simulink model "TCP"  (R2022b)
settings: Solver=FixedStepAuto  StartTime=0.0  StopTime=50000000  FixedStep=1  RelTol=1e-3
libraries: simulink x9
settings Model: Creator=yuzehong  LastModifiedBy=程一帆
settings OptimizationCC: DefaultParameterBehavior=Inlined  DefaultUnderspecifiedDataType=single  BufferReuse=off  GlobalBufferReuse=off  ExpressionFolding=off  EnableMemcpy=off  PassReuseOutputArgsAs=Individual arguments  OptimizeDataStoreBuffers=off  BusAssignmentInplaceUpdate=off  OptimizationLevel=level0  EfficientTunableParamExpr=on
settings DebuggingCC: ParameterTunabilityLossMsg=error  UnconnectedInputMsg=warning  UnconnectedOutputMsg=warning  UnconnectedLineMsg=warning
settings ModelReferenceCC: EnableRefExpFcnMdlSchedulingChecks=on
settings SFSimCC: MATLABDynamicMemAlloc=off
settings RTWCC: Description=Embedded Coder  SystemTargetFile=ert.tlc  GenCodeOnly=on  TemplateMakefile=ert_default_tmf  DLArmComputeVersion=19.05
settings CodeAppCC: ForceParamTrailComments=on  IgnoreCustomStorageClasses=off  OperatorAnnotations=on  SimulinkDataObjDesc=on  SFDataObjDesc=on  InsertBlockDesc=on
settings ERTTargetCC: TargetLangStandard=C99 (ISO)  GenerateSampleERTMain=on  CodeInterfacePackaging=Reusable function  InlinedParameterPlacement=NonHierarchical  ERTCustomFileTemplate=example_file_process.tlc
settings ConfigComp: DVMaxProcessTime=3600  DVTestSuiteOptimization=Auto  DVDetectOutOfBounds=on  DVSaveHarnessModel=on  DVModelReferenceHarness=on

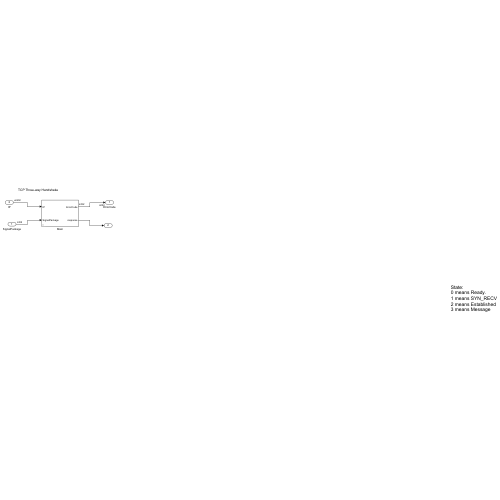
[thumbnail: Simulink's stored preview of the top-level diagram]
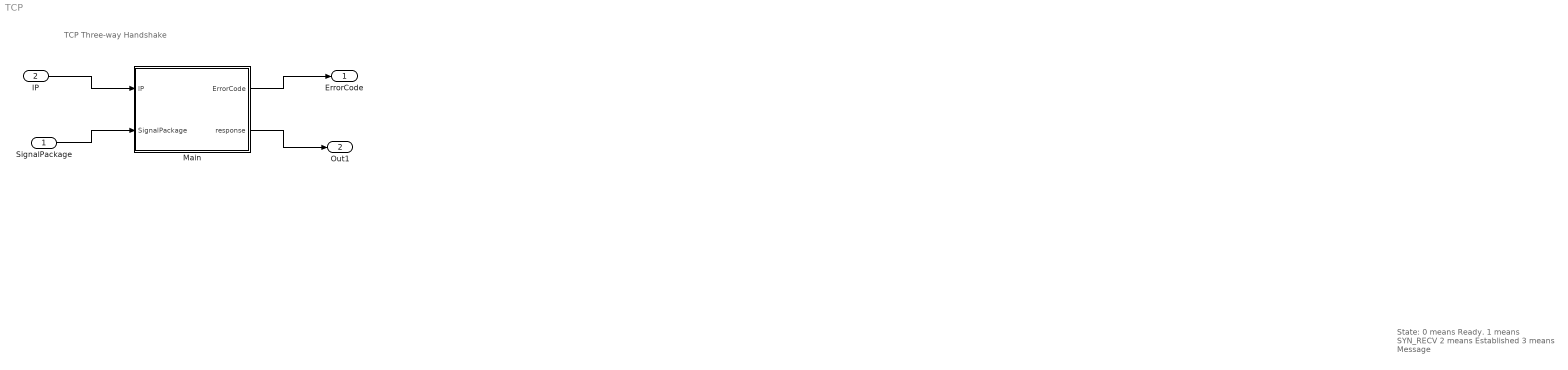
== system TCP ==
  note: TCP Three-way Handshake
  note: State:
      | 0 means Ready.
      | 1 means SYN_RECV
      | 2 means Established
      | 3 means Message
  SignalPackage : Inport  OutDataTypeStr=int32  PortDimensions=1
  IP : Inport  Port=2  OutDataTypeStr=uint32
  Main : Subsystem  mask{Len=16}
      mask DialogControl ParameterGroupVar Prompt: 参数
  ErrorCode : Outport  OutDataTypeStr=int32
  Out1 : Outport  Port=2
  wires:
  IP/1 -> Main/1(IP)
  SignalPackage/1 -> Main/2(SignalPackage)
  Main/1(ErrorCode) -> ErrorCode/1
  Main/2(response) -> Out1/1

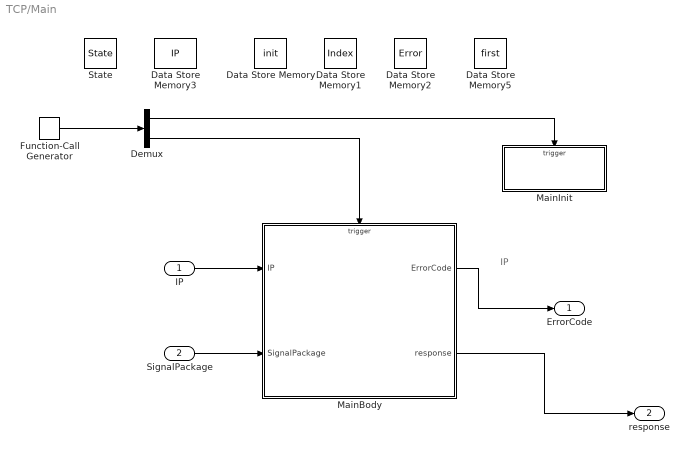
== system TCP/Main ==
  note: IP
  IP : Inport
  SignalPackage : Inport  Port=2
  Data Store Memory : DataStoreMemory  DataStoreName=init  WriteAfterWriteMsg=warning  ShowAdditionalParam=off  OutDataTypeStr=int8
  Data Store Memory1 : DataStoreMemory  DataStoreName=Index  WriteAfterWriteMsg=warning  InitialValue=-1  ShowAdditionalParam=off  OutDataTypeStr=int32
  Data Store Memory2 : DataStoreMemory  DataStoreName=Error  WriteAfterWriteMsg=warning  ShowAdditionalParam=off  OutDataTypeStr=int32
  Data Store Memory3 : DataStoreMemory  DataStoreName=IP  WriteAfterWriteMsg=warning  ShowAdditionalParam=off  OutDataTypeStr=uint32  Dimensions=Len
  Data Store Memory5 : DataStoreMemory  DataStoreName=first  WriteAfterWriteMsg=warning  ShowAdditionalParam=off  OutDataTypeStr=int32
  Demux : Demux  Outputs=2
  Function-Call Generator : simulink/Ports & Subsystems/Function-Call Generator  sample_time=1  numberOfIterations=1  DisallowWideOutput=off
  MainBody : Subsystem  TreatAsAtomicUnit=on
  MainInit : Subsystem  TreatAsAtomicUnit=on
  State : DataStoreMemory  DataStoreName=State  WriteAfterWriteMsg=warning  ShowAdditionalParam=off  OutDataTypeStr=int32  Dimensions=Len
  ErrorCode : Outport  OutDataTypeStr=int32
  response : Outport  Port=2
  wires:
  SignalPackage/1 -> MainBody/2(SignalPackage)
  Function-Call Generator/1 -> Demux/1
  Demux/1 -> MainInit/Trigger
  IP/1 -> MainBody/1(IP)
  MainBody/1(ErrorCode) -> ErrorCode/1
  Demux/2 -> MainBody/Trigger
  MainBody/2(response) -> response/1

== system TCP/Main/MainBody ==
  note: Process IP address.
  note: IP Address cannot be zero
  note: Process Data Package.
  IP : Inport
  SignalPackage : Inport  Port=2
  function : TriggerPort  TriggerType=function-call  VariantControl=(inherit)
  Process : Subsystem
  ErrorCode : Outport  OutDataTypeStr=int32
  response : Outport  Port=2
  wires:
  IP/1 -> Process/1(IP)
  SignalPackage/1 -> Process/2(SignalPackage)
  Process/1(ErrorCode) -> ErrorCode/1
  Process/2(response) -> response/1

== system TCP/Main/MainInit ==
  function : TriggerPort  TriggerType=function-call  VariantControl=(inherit)
  Data Store Read1 : DataStoreRead  DataStoreName=init  IndexOptions=Index vector (dialog)  Indices=1  OutputSizes=1
  If : If  IfExpression=u1 == 0
  If Action Subsystem : Subsystem  TreatAsAtomicUnit=on
  If Action Subsystem1 : Subsystem  TreatAsAtomicUnit=on
  wires:
  Data Store Read1/1 -> If/1
  If/1 -> If Action Subsystem/Action
  If/2 -> If Action Subsystem1/Action

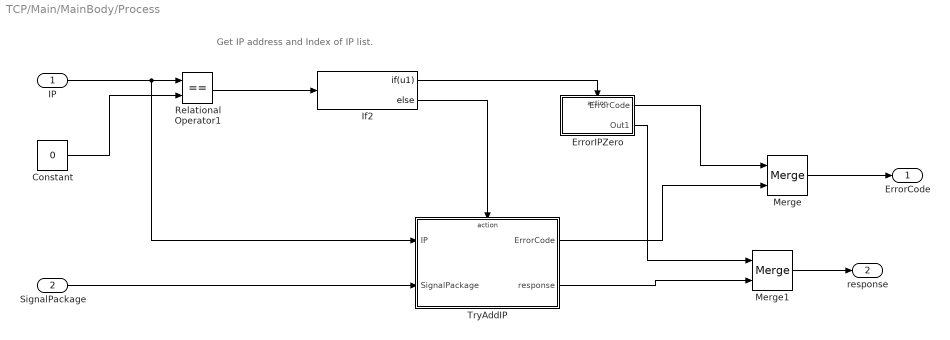
== system TCP/Main/MainBody/Process ==
  note: Get IP address and Index of IP list.
  IP : Inport
  SignalPackage : Inport  Port=2
  Constant : Constant  Value=0  OutDataTypeStr=uint32
  ErrorIPZero : Subsystem  TreatAsAtomicUnit=on
  If2 : If  IfExpression=u1
  Merge : Merge
  Merge1 : Merge
  Relational Operator1 : RelationalOperator  Operator===  OutDataTypeStr=boolean  InputSameDT=off
  TryAddIP : Subsystem  TreatAsAtomicUnit=on
  ErrorCode : Outport
  response : Outport  Port=2
  wires:
  If2/1 -> ErrorIPZero/Action
  If2/2 -> TryAddIP/Action
  Relational Operator1/1 -> If2/1
  Constant/1 -> Relational Operator1/2
  IP/1 -> TryAddIP/1(IP), Relational Operator1/1
  ErrorIPZero/1(ErrorCode) -> Merge/1
  TryAddIP/1(ErrorCode) -> Merge/2
  Merge/1 -> ErrorCode/1
  SignalPackage/1 -> TryAddIP/2(SignalPackage)
  TryAddIP/2(response) -> Merge1/2
  ErrorIPZero/2(Out1) -> Merge1/1
  Merge1/1 -> response/1

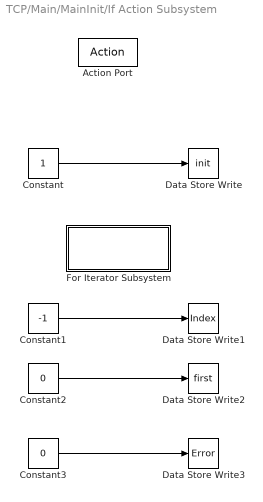
== system TCP/Main/MainInit/If Action Subsystem ==
  Action Port : ActionPort  ActionPortLabel=if(u1 == 0)
  Constant : Constant  OutDataTypeStr=int8
  Constant1 : Constant  Value=-1  OutDataTypeStr=int32
  Constant2 : Constant  Value=0  OutDataTypeStr=int32
  Constant3 : Constant  Value=0  OutDataTypeStr=int32
  Data Store Write : DataStoreWrite  DataStoreName=init  IndexOptions=Index vector (dialog)  Indices=1  OutputSizes=1
  Data Store Write1 : DataStoreWrite  DataStoreName=Index  IndexOptions=Index vector (dialog)  Indices=1  OutputSizes=1
  Data Store Write2 : DataStoreWrite  DataStoreName=first  IndexOptions=Index vector (dialog)  Indices=1  OutputSizes=1
  Data Store Write3 : DataStoreWrite  DataStoreName=Error  IndexOptions=Index vector (dialog)  Indices=1  OutputSizes=1
  For Iterator Subsystem : Subsystem  TreatAsAtomicUnit=on
  wires:
  Constant/1 -> Data Store Write/1
  Constant1/1 -> Data Store Write1/1
  Constant2/1 -> Data Store Write2/1
  Constant3/1 -> Data Store Write3/1

== system TCP/Main/MainInit/If Action Subsystem1 ==
  Action Port : ActionPort  ActionPortLabel=else
  Constant3 : Constant  Value=0  OutDataTypeStr=int32
  Data Store Write3 : DataStoreWrite  DataStoreName=Error  IndexOptions=Index vector (dialog)  Indices=1  OutputSizes=1
  wires:
  Constant3/1 -> Data Store Write3/1

== system TCP/Main/MainBody/Process/ErrorIPZero ==
  Action Port : ActionPort  ActionPortLabel=if(u1)
  Constant : Constant  OutDataTypeStr=int32
  Constant1 : Constant  OutDataTypeStr=int32
  Data Store Write : DataStoreWrite  DataStoreName=Error  IndexOptions=Index vector (dialog)  Indices=1  OutputSizes=1
  ErrorCode : Outport
  Out1 : Outport  Port=2
  wires:
  Constant/1 -> ErrorCode/1, Data Store Write/1
  Constant1/1 -> Out1/1

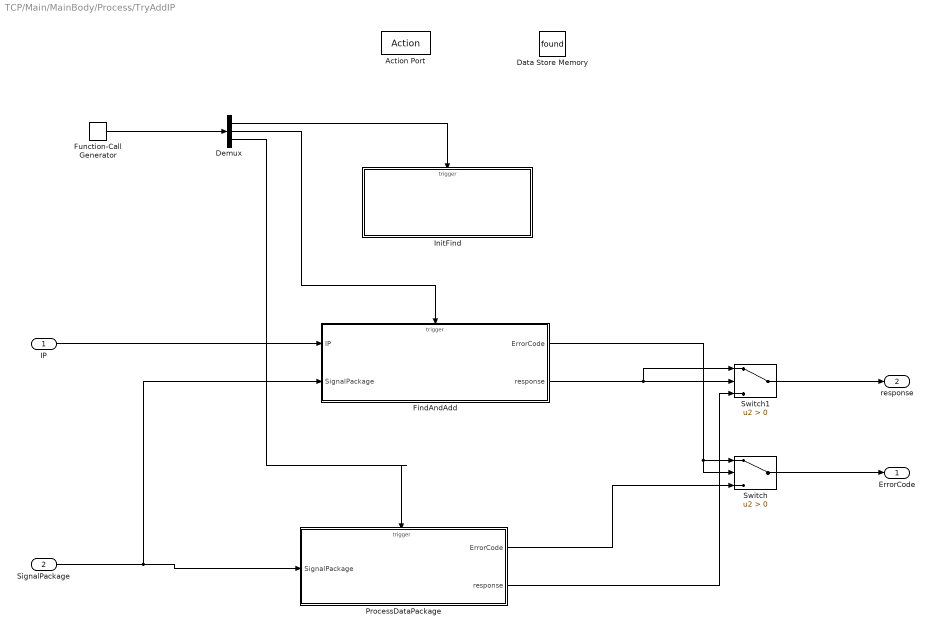
== system TCP/Main/MainBody/Process/TryAddIP ==
  IP : Inport
  SignalPackage : Inport  Port=2
  Action Port : ActionPort  ActionPortLabel=else
  Data Store Memory : DataStoreMemory  DataStoreName=found  WriteAfterWriteMsg=warning  InitialValue=-1  ShowAdditionalParam=off  OutDataTypeStr=int32
  Demux : Demux  Outputs=3
  FindAndAdd : Subsystem
  Function-Call Generator : simulink/Ports & Subsystems/Function-Call Generator  sample_time=-1  numberOfIterations=1  DisallowWideOutput=off
  InitFind : Subsystem
  ProcessDataPackage : Subsystem  TreatAsAtomicUnit=on
  Switch : Switch  Criteria=u2 > Threshold  SaturateOnIntegerOverflow=off  InputSameDT=off
  Switch1 : Switch  Criteria=u2 > Threshold  SaturateOnIntegerOverflow=off  InputSameDT=off
  ErrorCode : Outport
  response : Outport  Port=2
  wires:
  Demux/1 -> InitFind/Trigger
  IP/1 -> FindAndAdd/1(IP)
  Function-Call Generator/1 -> Demux/1
  Demux/2 -> FindAndAdd/Trigger
  SignalPackage/1 -> ProcessDataPackage/1(SignalPackage), FindAndAdd/2(SignalPackage)
  Demux/3 -> ProcessDataPackage/Trigger
  Switch/1 -> ErrorCode/1
  FindAndAdd/1(ErrorCode) -> Switch/1, Switch/2
  ProcessDataPackage/1(ErrorCode) -> Switch/3
  Switch1/1 -> response/1
  FindAndAdd/2(response) -> Switch1/1, Switch1/2
  ProcessDataPackage/2(response) -> Switch1/3

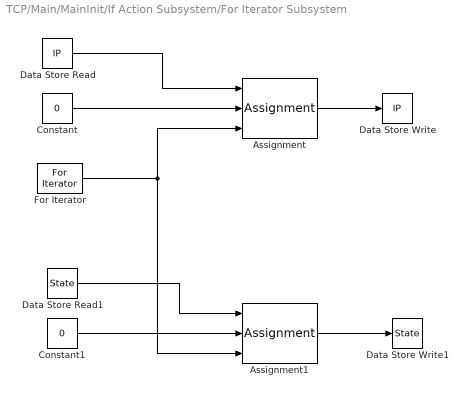
== system TCP/Main/MainInit/If Action Subsystem/For Iterator Subsystem ==
  Assignment : Assignment  IndexMode=Zero-based  DiagnosticForDimensions=Warning  IndexOptions=Index vector (port)  Indices=1  OutputSizes=1
  Assignment1 : Assignment  IndexMode=Zero-based  DiagnosticForDimensions=Warning  IndexOptions=Index vector (port)  Indices=1  OutputSizes=1
  Constant : Constant  Value=0  OutDataTypeStr=uint32
  Constant1 : Constant  Value=0  OutDataTypeStr=int32
  Data Store Read : DataStoreRead  DataStoreName=IP  IndexOptions=Index vector (dialog)  Indices=1  OutputSizes=1
  Data Store Read1 : DataStoreRead  DataStoreName=State  IndexOptions=Index vector (dialog)  Indices=1  OutputSizes=1
  Data Store Write : DataStoreWrite  DataStoreName=IP  IndexOptions=Index vector (dialog)  Indices=1  OutputSizes=1
  Data Store Write1 : DataStoreWrite  DataStoreName=State  IndexOptions=Index vector (dialog)  Indices=1  OutputSizes=1
  For Iterator : ForIterator  IterationLimit=Len  IndexMode=Zero-based
  wires:
  Data Store Read/1 -> Assignment/1
  For Iterator/1 -> Assignment1/3, Assignment/3
  Constant/1 -> Assignment/2
  Assignment/1 -> Data Store Write/1
  Assignment1/1 -> Data Store Write1/1
  Constant1/1 -> Assignment1/2
  Data Store Read1/1 -> Assignment1/1

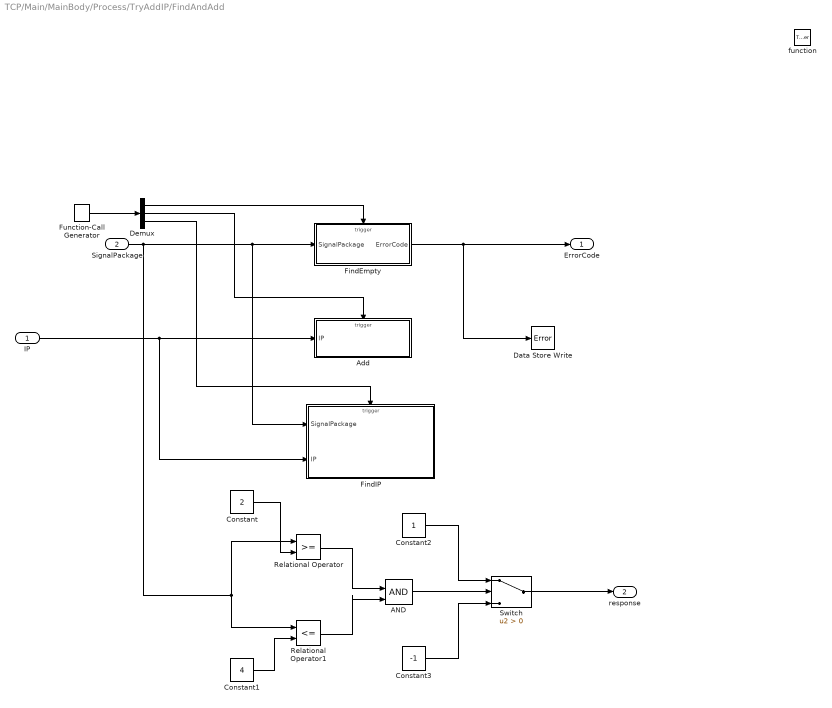
== system TCP/Main/MainBody/Process/TryAddIP/FindAndAdd ==
  IP : Inport
  SignalPackage : Inport  Port=2
  function : TriggerPort  TriggerType=function-call  VariantControl=(inherit)
  AND : Logic  IconShape=distinctive  AllPortsSameDT=off  OutDataTypeStr=boolean
  Add : Subsystem
  Constant : Constant  Value=2  OutDataTypeStr=int32
  Constant1 : Constant  Value=4  OutDataTypeStr=int32
  Constant2 : Constant  OutDataTypeStr=int32
  Constant3 : Constant  Value=-1  OutDataTypeStr=int32
  Data Store Write : DataStoreWrite  DataStoreName=Error  IndexOptions=Index vector (dialog)  Indices=1  OutputSizes=1
  Demux : Demux  Outputs=3
  FindEmpty : Subsystem
  FindIP : Subsystem
  Function-Call Generator : simulink/Ports & Subsystems/Function-Call Generator  sample_time=-1  numberOfIterations=1  DisallowWideOutput=off
  Relational Operator : RelationalOperator  OutDataTypeStr=boolean  RndMeth=Simplest  InputSameDT=off
  Relational Operator1 : RelationalOperator  Operator=<=  OutDataTypeStr=boolean  RndMeth=Simplest  InputSameDT=off
  Switch : Switch  Criteria=u2 > Threshold  SaturateOnIntegerOverflow=off  InputSameDT=off
  ErrorCode : Outport
  response : Outport  Port=2
  wires:
  Function-Call Generator/1 -> Demux/1
  IP/1 -> FindIP/2(IP), Add/1(IP)
  Demux/2 -> Add/Trigger
  Demux/1 -> FindEmpty/Trigger
  FindEmpty/1(ErrorCode) -> Data Store Write/1, ErrorCode/1
  Demux/3 -> FindIP/Trigger
  Relational Operator1/1 -> AND/2
  AND/1 -> Switch/2
  Constant/1 -> Relational Operator/2
  Constant2/1 -> Switch/1
  Relational Operator/1 -> AND/1
  Constant1/1 -> Relational Operator1/2
  Constant3/1 -> Switch/3
  SignalPackage/1 -> FindEmpty/1(SignalPackage), FindIP/1(SignalPackage), Relational Operator/1, Relational Operator1/1
  Switch/1 -> response/1

== system TCP/Main/MainBody/Process/TryAddIP/InitFind ==
  function : TriggerPort  TriggerType=function-call  VariantControl=(inherit)
  Constant1 : Constant  Value=-1  OutDataTypeStr=int32
  Constant2 : Constant  Value=-1  OutDataTypeStr=int32
  Data Store Write1 : DataStoreWrite  DataStoreName=found  IndexOptions=Index vector (dialog)  Indices=1  OutputSizes=1
  Data Store Write2 : DataStoreWrite  DataStoreName=Index  IndexOptions=Index vector (dialog)  Indices=1  OutputSizes=1
  wires:
  Constant1/1 -> Data Store Write1/1
  Constant2/1 -> Data Store Write2/1

== system TCP/Main/MainBody/Process/TryAddIP/ProcessDataPackage ==
  note: State:
      | 0 means Ready.
      | 1 means SYN_RECV.
      | 2 means Established.
  note: Signal:
      | 0 means SYN.
      | 1 means ACK.
      | 2 means Message.
  SignalPackage : Inport
  function : TriggerPort  TriggerType=function-call  VariantControl=(inherit)
  BeginHandShake : Subsystem  TreatAsAtomicUnit=on
  Compare To Constant : simulink/Logic and Bit Operations/Compare To Constant  relop=~=  const=-1  OutDataTypeStr=boolean
  Data Store Read2 : DataStoreRead  DataStoreName=Index  IndexOptions=Index vector (dialog)  Indices=1  OutputSizes=1
  If : If  IfExpression=u1 ~= 0
  Terminator : Terminator
  ErrorCode : Outport  OutDataTypeStr=int32
  response : Outport  Port=2
  wires:
  Data Store Read2/1 -> Compare To Constant/1
  Compare To Constant/1 -> If/1
  If/1 -> BeginHandShake/Action
  If/2 -> Terminator/1
  SignalPackage/1 -> BeginHandShake/1(SignalPackage)
  BeginHandShake/1(ErrorCode) -> ErrorCode/1
  BeginHandShake/2(response) -> response/1

== system TCP/Main/MainBody/Process/TryAddIP/FindAndAdd/Add ==
  IP : Inport
  function : TriggerPort  TriggerType=function-call  VariantControl=(inherit)
  Add : Subsystem  TreatAsAtomicUnit=on
  Compare To Constant : simulink/Logic and Bit Operations/Compare To Constant  relop===  const=-1  OutDataTypeStr=boolean
  Data Store Read1 : DataStoreRead  DataStoreName=found  IndexOptions=Index vector (dialog)  Indices=1  OutputSizes=1
  If : If  IfExpression=u1 ~= 0
  Terminator : Terminator
  wires:
  If/2 -> Add/Action
  Data Store Read1/1 -> Add/2(index), Compare To Constant/1
  Compare To Constant/1 -> If/1
  If/1 -> Terminator/1
  IP/1 -> Add/1(IP)

== system TCP/Main/MainBody/Process/TryAddIP/FindAndAdd/FindEmpty ==
  SignalPackage : Inport
  function : TriggerPort  TriggerType=function-call  VariantControl=(inherit)
  Compare To Constant : simulink/Logic and Bit Operations/Compare To Constant  relop===  const=0  OutDataTypeStr=boolean
  ErrorSignal : Subsystem  TreatAsAtomicUnit=on
  FindEmpty : Subsystem
  If : If  IfExpression=u1 ~= 0
  Merge : Merge
  ErrorCode : Outport
  wires:
  SignalPackage/1 -> Compare To Constant/1
  Compare To Constant/1 -> If/1
  ErrorSignal/1(ErrorCode) -> Merge/1
  Merge/1 -> ErrorCode/1
  If/2 -> ErrorSignal/Action
  FindEmpty/1(ErrorCode) -> Merge/2
  If/1 -> FindEmpty/Action

== system TCP/Main/MainBody/Process/TryAddIP/FindAndAdd/FindIP ==
  SignalPackage : Inport
  IP : Inport  Port=2
  function : TriggerPort  TriggerType=function-call  VariantControl=(inherit)
  Compare To Constant : simulink/Logic and Bit Operations/Compare To Constant  relop=~=  const=0  OutDataTypeStr=boolean
  FindEmpty : Subsystem
  If : If  IfExpression=u1 ~= 0
  Terminator : Terminator
  wires:
  SignalPackage/1 -> Compare To Constant/1
  If/1 -> FindEmpty/Action
  If/2 -> Terminator/1
  IP/1 -> FindEmpty/1(IP)
  Compare To Constant/1 -> If/1

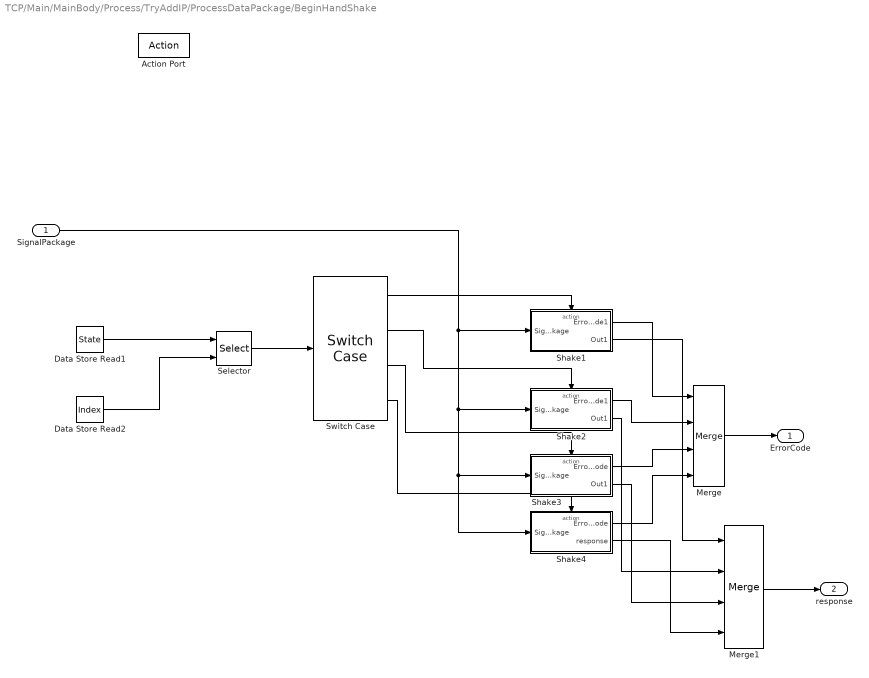
== system TCP/Main/MainBody/Process/TryAddIP/ProcessDataPackage/BeginHandShake ==
  SignalPackage : Inport
  Action Port : ActionPort  ActionPortLabel=if(u1 ~= 0)
  Data Store Read1 : DataStoreRead  DataStoreName=State  IndexOptions=Index vector (dialog)  Indices=1  OutputSizes=1
  Data Store Read2 : DataStoreRead  DataStoreName=Index  IndexOptions=Index vector (dialog)  Indices=1  OutputSizes=1
  Merge : Merge  Inputs=4
  Merge1 : Merge  Inputs=4
  Selector : Selector  IndexMode=Zero-based  InputPortWidth=Len  IndexOptions=Index vector (port)  Indices=[1 3]  OutputSizes=1
  Shake1 : Subsystem  TreatAsAtomicUnit=on
  Shake2 : Subsystem  TreatAsAtomicUnit=on
  Shake3 : Subsystem  TreatAsAtomicUnit=on
  Shake4 : Subsystem  TreatAsAtomicUnit=on
  Switch Case : SwitchCase  CaseConditions={1,2,3}
  ErrorCode : Outport
  response : Outport  Port=2
  wires:
  Data Store Read1/1 -> Selector/1
  Merge/1 -> ErrorCode/1
  Switch Case/2 -> Shake2/Action
  SignalPackage/1 -> Shake4/1(SignalPackage), Shake3/1(SignalPackage), Shake2/1(SignalPackage), Shake1/1(SignalPackage)
  Selector/1 -> Switch Case/1
  Switch Case/1 -> Shake1/Action
  Switch Case/3 -> Shake3/Action
  Shake3/1(ErrorCode) -> Merge/3
  Data Store Read2/1 -> Selector/2
  Shake1/1(ErrorCode1) -> Merge/1
  Shake2/1(ErrorCode1) -> Merge/2
  Shake4/1(ErrorCode) -> Merge/4
  Switch Case/4 -> Shake4/Action
  Shake4/2(response) -> Merge1/4
  Merge1/1 -> response/1
  Shake3/2(Out1) -> Merge1/3
  Shake2/2(Out1) -> Merge1/2
  Shake1/2(Out1) -> Merge1/1

== system TCP/Main/MainBody/Process/TryAddIP/FindAndAdd/Add/Add ==
  IP : Inport
  index : Inport  Port=2
  Action Port : ActionPort  ActionPortLabel=else
  ForAdd : Subsystem  TreatAsAtomicUnit=on
  wires:
  IP/1 -> ForAdd/1(IP)
  index/1 -> ForAdd/2(index)

== system TCP/Main/MainBody/Process/TryAddIP/FindAndAdd/FindEmpty/ErrorSignal ==
  Action Port : ActionPort  ActionPortLabel=else
  Constant : Constant  Value=2  OutDataTypeStr=int32
  ErrorCode : Outport
  wires:
  Constant/1 -> ErrorCode/1

== system TCP/Main/MainBody/Process/TryAddIP/FindAndAdd/FindEmpty/FindEmpty ==
  Action Port : ActionPort  ActionPortLabel=if(u1 ~= 0)
  ForFind : Subsystem  TreatAsAtomicUnit=on
  ErrorCode : Outport
  wires:
  ForFind/1(ErrorCode) -> ErrorCode/1

== system TCP/Main/MainBody/Process/TryAddIP/FindAndAdd/FindIP/FindEmpty ==
  IP : Inport
  Action Port : ActionPort  ActionPortLabel=if(u1 ~= 0)
  ForFind : Subsystem  TreatAsAtomicUnit=on
  wires:
  IP/1 -> ForFind/1(IP)

== system TCP/Main/MainBody/Process/TryAddIP/ProcessDataPackage/BeginHandShake/Shake1 ==
  SignalPackage : Inport
  Action Port : ActionPort  ActionPortLabel=case [ 1 ]:
  Constant1 : Constant  OutDataTypeStr=int32
  If : If  IfExpression=u1 == 0
  If Action Subsystem : Subsystem  TreatAsAtomicUnit=on
  If Action Subsystem1 : Subsystem  TreatAsAtomicUnit=on
  Merge : Merge
  ErrorCode1 : Outport  OutDataTypeStr=int32
  Out1 : Outport  Port=2
  wires:
  If/2 -> If Action Subsystem1/Action
  If Action Subsystem/1(ErrorCode) -> Merge/1
  SignalPackage/1 -> If/1
  If/1 -> If Action Subsystem/Action
  Constant1/1 -> Out1/1
  If Action Subsystem1/1(Out1) -> Merge/2
  Merge/1 -> ErrorCode1/1

== system TCP/Main/MainBody/Process/TryAddIP/ProcessDataPackage/BeginHandShake/Shake2 ==
  SignalPackage : Inport
  Action Port : ActionPort  ActionPortLabel=case [ 2 ]:
  Constant1 : Constant  OutDataTypeStr=int32
  If : If  IfExpression=u1 == 2
  If Action Subsystem : Subsystem  TreatAsAtomicUnit=on
  If Action Subsystem1 : Subsystem  TreatAsAtomicUnit=on
  Merge : Merge
  ErrorCode1 : Outport  OutDataTypeStr=int32
  Out1 : Outport  Port=2
  wires:
  SignalPackage/1 -> If/1
  If Action Subsystem/1(ErrorCode) -> Merge/1
  If/2 -> If Action Subsystem1/Action
  If/1 -> If Action Subsystem/Action
  Constant1/1 -> Out1/1
  If Action Subsystem1/1(Out1) -> Merge/2
  Merge/1 -> ErrorCode1/1

== system TCP/Main/MainBody/Process/TryAddIP/ProcessDataPackage/BeginHandShake/Shake3 ==
  SignalPackage : Inport
  Action Port : ActionPort  ActionPortLabel=case [ 3 ]:
  Constant1 : Constant  OutDataTypeStr=int32
  If : If  IfExpression=u1 == 3
  If Action Subsystem : Subsystem  TreatAsAtomicUnit=on
  If Action Subsystem1 : Subsystem  TreatAsAtomicUnit=on
  Merge : Merge
  ErrorCode : Outport  OutDataTypeStr=int32
  Out1 : Outport  Port=2
  wires:
  SignalPackage/1 -> If/1
  If/1 -> If Action Subsystem/Action
  If Action Subsystem/1(ErrorCode) -> Merge/1
  Constant1/1 -> Out1/1
  If/2 -> If Action Subsystem1/Action
  If Action Subsystem1/1(Out1) -> Merge/2
  Merge/1 -> ErrorCode/1

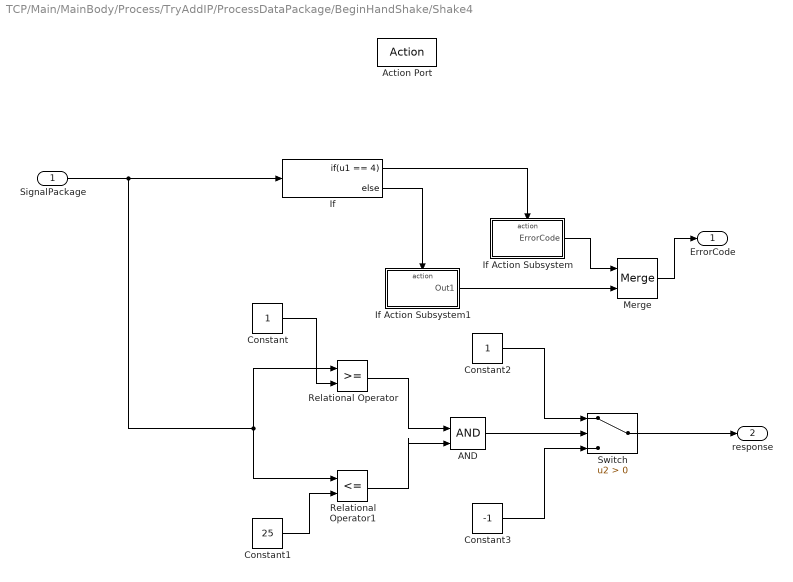
== system TCP/Main/MainBody/Process/TryAddIP/ProcessDataPackage/BeginHandShake/Shake4 ==
  SignalPackage : Inport
  Action Port : ActionPort  ActionPortLabel=default:
  AND : Logic  IconShape=distinctive  AllPortsSameDT=off  OutDataTypeStr=boolean
  Constant : Constant  OutDataTypeStr=int32
  Constant1 : Constant  Value=25  OutDataTypeStr=int32
  Constant2 : Constant  OutDataTypeStr=int32
  Constant3 : Constant  Value=-1  OutDataTypeStr=int32
  If : If  IfExpression=u1 == 4
  If Action Subsystem : Subsystem  TreatAsAtomicUnit=on
  If Action Subsystem1 : Subsystem  TreatAsAtomicUnit=on
  Merge : Merge
  Relational Operator : RelationalOperator  OutDataTypeStr=boolean  RndMeth=Simplest  InputSameDT=off
  Relational Operator1 : RelationalOperator  Operator=<=  OutDataTypeStr=boolean  RndMeth=Simplest  InputSameDT=off
  Switch : Switch  Criteria=u2 > Threshold  SaturateOnIntegerOverflow=off  InputSameDT=off
  ErrorCode : Outport  OutDataTypeStr=int32
  response : Outport  Port=2
  wires:
  If/1 -> If Action Subsystem/Action
  Relational Operator1/1 -> AND/2
  AND/1 -> Switch/2
  Constant/1 -> Relational Operator/2
  Constant2/1 -> Switch/1
  Relational Operator/1 -> AND/1
  Constant1/1 -> Relational Operator1/2
  Constant3/1 -> Switch/3
  SignalPackage/1 -> Relational Operator/1, Relational Operator1/1, If/1
  Switch/1 -> response/1
  If/2 -> If Action Subsystem1/Action
  If Action Subsystem/1(ErrorCode) -> Merge/1
  If Action Subsystem1/1(Out1) -> Merge/2
  Merge/1 -> ErrorCode/1

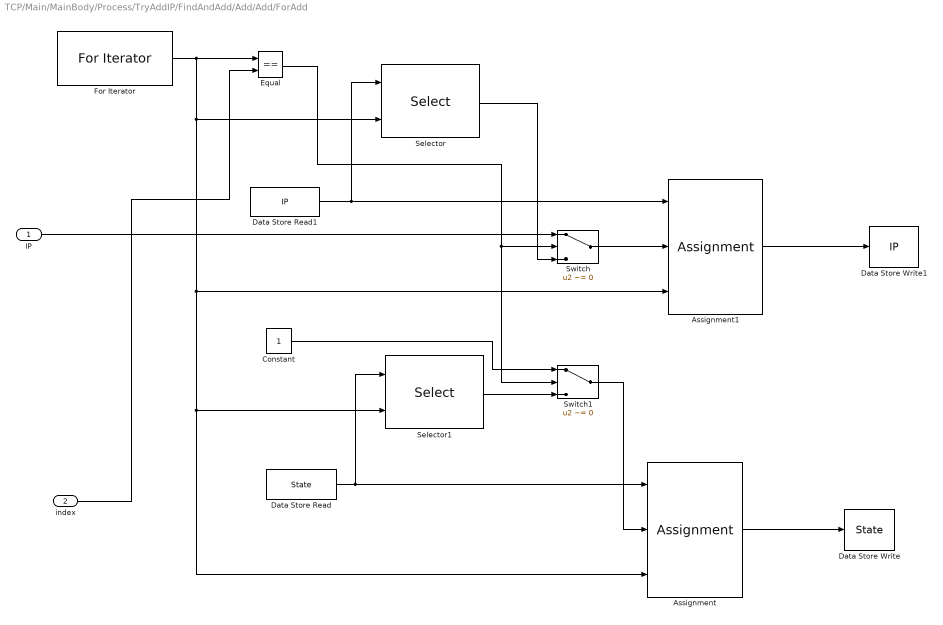
== system TCP/Main/MainBody/Process/TryAddIP/FindAndAdd/Add/Add/ForAdd ==
  IP : Inport
  index : Inport  Port=2
  Assignment : Assignment  IndexMode=Zero-based  DiagnosticForDimensions=Warning  IndexOptions=Index vector (port)  Indices=1  OutputSizes=1
  Assignment1 : Assignment  IndexMode=Zero-based  DiagnosticForDimensions=Warning  IndexOptions=Index vector (port)  Indices=1  OutputSizes=1
  Constant : Constant  OutDataTypeStr=int32
  Data Store Read : DataStoreRead  DataStoreName=State  IndexOptions=Index vector (dialog)  Indices=1  OutputSizes=1
  Data Store Read1 : DataStoreRead  DataStoreName=IP  IndexOptions=Index vector (dialog)  Indices=1  OutputSizes=1
  Data Store Write : DataStoreWrite  DataStoreName=State  IndexOptions=Index vector (dialog)  Indices=1  OutputSizes=1
  Data Store Write1 : DataStoreWrite  DataStoreName=IP  IndexOptions=Index vector (dialog)  Indices=1  OutputSizes=1
  Equal : RelationalOperator  Operator===  OutDataTypeStr=boolean  RndMeth=Simplest  InputSameDT=off
  For Iterator : ForIterator  IterationLimit=Len  IndexMode=Zero-based
  Selector : Selector  IndexMode=Zero-based  InputPortWidth=Len  IndexOptions=Index vector (port)  Indices=[1 3]  OutputSizes=1
  Selector1 : Selector  IndexMode=Zero-based  InputPortWidth=Len  IndexOptions=Index vector (port)  Indices=[1 3]  OutputSizes=1
  Switch : Switch  Criteria=u2 ~= 0  SaturateOnIntegerOverflow=off  InputSameDT=off
  Switch1 : Switch  Criteria=u2 ~= 0  SaturateOnIntegerOverflow=off  InputSameDT=off
  wires:
  Data Store Read1/1 -> Selector/1, Assignment1/1
  Assignment/1 -> Data Store Write/1
  Assignment1/1 -> Data Store Write1/1
  For Iterator/1 -> Assignment1/3, Assignment/3, Selector1/2, Selector/2, Equal/1
  index/1 -> Equal/2
  Data Store Read/1 -> Selector1/1, Assignment/1
  Equal/1 -> Switch1/2, Switch/2
  IP/1 -> Switch/1
  Switch/1 -> Assignment1/2
  Selector/1 -> Switch/3
  Selector1/1 -> Switch1/3
  Constant/1 -> Switch1/1
  Switch1/1 -> Assignment/2

== system TCP/Main/MainBody/Process/TryAddIP/FindAndAdd/FindEmpty/FindEmpty/ForFind ==
  Constant : Constant  Value=0  OutDataTypeStr=int32
  Data Store Read1 : DataStoreRead  DataStoreName=State  IndexOptions=Index vector (dialog)  Indices=1  OutputSizes=1
  ExistEmptyPlace : Subsystem  TreatAsAtomicUnit=on
  For Iterator : ForIterator  IterationLimit=Len  IndexMode=Zero-based
  If : If  IfExpression=u1
  Relational Operator : RelationalOperator  Operator===  OutDataTypeStr=boolean  RndMeth=Simplest  InputSameDT=off
  Selector : Selector  IndexMode=Zero-based  InputPortWidth=Len  IndexOptions=Index vector (port)  Indices=[1 3]  OutputSizes=1
  Terminator : Terminator
  ErrorCode : Outport
  wires:
  For Iterator/1 -> ExistEmptyPlace/1(Index), Selector/2
  Data Store Read1/1 -> Selector/1
  Selector/1 -> Relational Operator/1
  Constant/1 -> ErrorCode/1, Relational Operator/2
  If/1 -> ExistEmptyPlace/Action
  Relational Operator/1 -> If/1
  If/2 -> Terminator/1

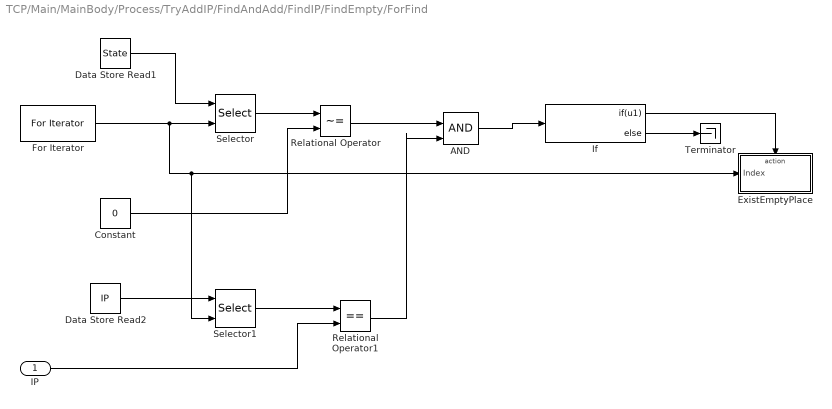
== system TCP/Main/MainBody/Process/TryAddIP/FindAndAdd/FindIP/FindEmpty/ForFind ==
  IP : Inport
  AND : Logic  IconShape=distinctive  AllPortsSameDT=off  OutDataTypeStr=boolean
  Constant : Constant  Value=0  OutDataTypeStr=int32
  Data Store Read1 : DataStoreRead  DataStoreName=State  IndexOptions=Index vector (dialog)  Indices=1  OutputSizes=1
  Data Store Read2 : DataStoreRead  DataStoreName=IP  IndexOptions=Index vector (dialog)  Indices=1  OutputSizes=1
  ExistEmptyPlace : Subsystem  TreatAsAtomicUnit=on
  For Iterator : ForIterator  IterationLimit=Len  IndexMode=Zero-based
  If : If  IfExpression=u1
  Relational Operator : RelationalOperator  Operator=~=  OutDataTypeStr=boolean  RndMeth=Simplest  InputSameDT=off
  Relational Operator1 : RelationalOperator  Operator===  OutDataTypeStr=boolean  RndMeth=Simplest  InputSameDT=off
  Selector : Selector  IndexMode=Zero-based  InputPortWidth=Len  IndexOptions=Index vector (port)  Indices=[1 3]  OutputSizes=1
  Selector1 : Selector  IndexMode=Zero-based  InputPortWidth=Len  IndexOptions=Index vector (port)  Indices=[1 3]  OutputSizes=1
  Terminator : Terminator
  wires:
  For Iterator/1 -> Selector1/2, ExistEmptyPlace/1(Index), Selector/2
  Data Store Read1/1 -> Selector/1
  Selector/1 -> Relational Operator/1
  Constant/1 -> Relational Operator/2
  If/1 -> ExistEmptyPlace/Action
  Relational Operator/1 -> AND/1
  If/2 -> Terminator/1
  Data Store Read2/1 -> Selector1/1
  Selector1/1 -> Relational Operator1/1
  IP/1 -> Relational Operator1/2
  Relational Operator1/1 -> AND/2
  AND/1 -> If/1

== system TCP/Main/MainBody/Process/TryAddIP/ProcessDataPackage/BeginHandShake/Shake1/If Action Subsystem ==
  Action Port : ActionPort  ActionPortLabel=if(u1 == 0)
  Constant1 : Constant  Value=0  OutDataTypeStr=int32
  Data Store Read2 : DataStoreRead  DataStoreName=Index  IndexOptions=Index vector (dialog)  Indices=1  OutputSizes=1
  For Iterator Subsystem : Subsystem  TreatAsAtomicUnit=on
  ErrorCode : Outport
  wires:
  Constant1/1 -> ErrorCode/1
  Data Store Read2/1 -> For Iterator Subsystem/1(index)

== system TCP/Main/MainBody/Process/TryAddIP/ProcessDataPackage/BeginHandShake/Shake1/If Action Subsystem1 ==
  Action Port : ActionPort  ActionPortLabel=else
  Constant1 : Constant  OutDataTypeStr=int32
  Out1 : Outport
  wires:
  Constant1/1 -> Out1/1

== system TCP/Main/MainBody/Process/TryAddIP/ProcessDataPackage/BeginHandShake/Shake2/If Action Subsystem ==
  Action Port : ActionPort  ActionPortLabel=if(u1 == 2)
  Constant1 : Constant  Value=0  OutDataTypeStr=int32
  Data Store Read2 : DataStoreRead  DataStoreName=Index  IndexOptions=Index vector (dialog)  Indices=1  OutputSizes=1
  For Iterator Subsystem : Subsystem  TreatAsAtomicUnit=on
  ErrorCode : Outport
  wires:
  Constant1/1 -> ErrorCode/1
  Data Store Read2/1 -> For Iterator Subsystem/1(index)

== system TCP/Main/MainBody/Process/TryAddIP/ProcessDataPackage/BeginHandShake/Shake2/If Action Subsystem1 ==
  Action Port : ActionPort  ActionPortLabel=else
  Constant1 : Constant  OutDataTypeStr=int32
  Out1 : Outport
  wires:
  Constant1/1 -> Out1/1

== system TCP/Main/MainBody/Process/TryAddIP/ProcessDataPackage/BeginHandShake/Shake3/If Action Subsystem ==
  Action Port : ActionPort  ActionPortLabel=if(u1 == 3)
  Constant1 : Constant  Value=0  OutDataTypeStr=int32
  Data Store Read2 : DataStoreRead  DataStoreName=Index  IndexOptions=Index vector (dialog)  Indices=1  OutputSizes=1
  For Iterator Subsystem : Subsystem  TreatAsAtomicUnit=on
  ErrorCode : Outport
  wires:
  Constant1/1 -> ErrorCode/1
  Data Store Read2/1 -> For Iterator Subsystem/1(index)

== system TCP/Main/MainBody/Process/TryAddIP/ProcessDataPackage/BeginHandShake/Shake3/If Action Subsystem1 ==
  Action Port : ActionPort  ActionPortLabel=else
  Constant1 : Constant  OutDataTypeStr=int32
  Out1 : Outport
  wires:
  Constant1/1 -> Out1/1

== system TCP/Main/MainBody/Process/TryAddIP/ProcessDataPackage/BeginHandShake/Shake4/If Action Subsystem ==
  Action Port : ActionPort  ActionPortLabel=if(u1 == 4)
  Constant1 : Constant  Value=0  OutDataTypeStr=int32
  Data Store Read2 : DataStoreRead  DataStoreName=Index  IndexOptions=Index vector (dialog)  Indices=1  OutputSizes=1
  For Iterator Subsystem : Subsystem  TreatAsAtomicUnit=on
  ErrorCode : Outport
  wires:
  Constant1/1 -> ErrorCode/1
  Data Store Read2/1 -> For Iterator Subsystem/1(index)

== system TCP/Main/MainBody/Process/TryAddIP/ProcessDataPackage/BeginHandShake/Shake4/If Action Subsystem1 ==
  Action Port : ActionPort  ActionPortLabel=else
  Constant1 : Constant  OutDataTypeStr=int32
  Out1 : Outport
  wires:
  Constant1/1 -> Out1/1

== system TCP/Main/MainBody/Process/TryAddIP/FindAndAdd/FindEmpty/FindEmpty/ForFind/ExistEmptyPlace ==
  Index : Inport
  Action Port : ActionPort  ActionPortLabel=if(u1)
  Compare To Constant : simulink/Logic and Bit Operations/Compare To Constant  relop===  const=-1  OutDataTypeStr=boolean
  Data Store Read : DataStoreRead  DataStoreName=found  IndexOptions=Index vector (dialog)  Indices=1  OutputSizes=1
  Data Store Write : DataStoreWrite  DataStoreName=found  IndexOptions=Index vector (dialog)  Indices=1  OutputSizes=1
  Data Store Write1 : DataStoreWrite  DataStoreName=Index  IndexOptions=Index vector (dialog)  Indices=1  OutputSizes=1
  Display : Display
  Display1 : Display
  Switch : Switch  Criteria=u2 > Threshold  SaturateOnIntegerOverflow=off  InputSameDT=off
  wires:
  Data Store Read/1 -> Display1/1, Switch/3, Compare To Constant/1
  Compare To Constant/1 -> Switch/2
  Index/1 -> Switch/1
  Switch/1 -> Data Store Write1/1, Display/1, Data Store Write/1

== system TCP/Main/MainBody/Process/TryAddIP/FindAndAdd/FindIP/FindEmpty/ForFind/ExistEmptyPlace ==
  Index : Inport
  Action Port : ActionPort  ActionPortLabel=if(u1)
  Compare To Constant : simulink/Logic and Bit Operations/Compare To Constant  relop===  const=-1  OutDataTypeStr=boolean
  Data Store Read1 : DataStoreRead  DataStoreName=Index  IndexOptions=Index vector (dialog)  Indices=1  OutputSizes=1
  Data Store Write1 : DataStoreWrite  DataStoreName=Index  IndexOptions=Index vector (dialog)  Indices=1  OutputSizes=1
  Switch : Switch  Criteria=u2 > Threshold  SaturateOnIntegerOverflow=off  InputSameDT=off
  wires:
  Data Store Read1/1 -> Switch/3, Compare To Constant/1
  Compare To Constant/1 -> Switch/2
  Index/1 -> Switch/1
  Switch/1 -> Data Store Write1/1

== system TCP/Main/MainBody/Process/TryAddIP/ProcessDataPackage/BeginHandShake/Shake1/If Action Subsystem/For Iterator Subsystem ==
  index : Inport
  Assignment : Assignment  IndexMode=Zero-based  DiagnosticForDimensions=Warning  IndexOptions=Index vector (port)  Indices=1  OutputSizes=1
  Constant : Constant  Value=2  OutDataTypeStr=int32
  Data Store Read1 : DataStoreRead  DataStoreName=State  IndexOptions=Index vector (dialog)  Indices=1  OutputSizes=1
  Data Store Write : DataStoreWrite  DataStoreName=State  IndexOptions=Index vector (dialog)  Indices=1  OutputSizes=1
  Equal : RelationalOperator  Operator===  OutDataTypeStr=boolean  RndMeth=Simplest  InputSameDT=off
  For Iterator : ForIterator  IterationLimit=Len  IndexMode=Zero-based
  Selector : Selector  IndexMode=Zero-based  InputPortWidth=Len  IndexOptions=Index vector (port)  Indices=[1 3]  OutputSizes=1
  Switch : Switch  Criteria=u2 ~= 0  SaturateOnIntegerOverflow=off  InputSameDT=off
  wires:
  Assignment/1 -> Data Store Write/1
  For Iterator/1 -> Selector/2, Assignment/3, Equal/1
  index/1 -> Equal/2
  Data Store Read1/1 -> Assignment/1, Selector/1
  Constant/1 -> Switch/1
  Equal/1 -> Switch/2
  Selector/1 -> Switch/3
  Switch/1 -> Assignment/2

== system TCP/Main/MainBody/Process/TryAddIP/ProcessDataPackage/BeginHandShake/Shake2/If Action Subsystem/For Iterator Subsystem ==
  index : Inport
  Assignment : Assignment  IndexMode=Zero-based  DiagnosticForDimensions=Warning  IndexOptions=Index vector (port)  Indices=1  OutputSizes=1
  Constant : Constant  Value=3  OutDataTypeStr=int32
  Data Store Read1 : DataStoreRead  DataStoreName=State  IndexOptions=Index vector (dialog)  Indices=1  OutputSizes=1
  Data Store Write : DataStoreWrite  DataStoreName=State  IndexOptions=Index vector (dialog)  Indices=1  OutputSizes=1
  Equal : RelationalOperator  Operator===  OutDataTypeStr=boolean  RndMeth=Simplest  InputSameDT=off
  For Iterator : ForIterator  IterationLimit=Len  IndexMode=Zero-based
  Selector : Selector  IndexMode=Zero-based  InputPortWidth=Len  IndexOptions=Index vector (port)  Indices=[1 3]  OutputSizes=1
  Switch : Switch  Criteria=u2 ~= 0  SaturateOnIntegerOverflow=off  InputSameDT=off
  wires:
  Assignment/1 -> Data Store Write/1
  For Iterator/1 -> Selector/2, Assignment/3, Equal/1
  index/1 -> Equal/2
  Data Store Read1/1 -> Assignment/1, Selector/1
  Constant/1 -> Switch/1
  Equal/1 -> Switch/2
  Selector/1 -> Switch/3
  Switch/1 -> Assignment/2

== system TCP/Main/MainBody/Process/TryAddIP/ProcessDataPackage/BeginHandShake/Shake3/If Action Subsystem/For Iterator Subsystem ==
  index : Inport
  Assignment : Assignment  IndexMode=Zero-based  DiagnosticForDimensions=Warning  IndexOptions=Index vector (port)  Indices=1  OutputSizes=1
  Constant : Constant  Value=4  OutDataTypeStr=int32
  Data Store Read1 : DataStoreRead  DataStoreName=State  IndexOptions=Index vector (dialog)  Indices=1  OutputSizes=1
  Data Store Write : DataStoreWrite  DataStoreName=State  IndexOptions=Index vector (dialog)  Indices=1  OutputSizes=1
  Equal : RelationalOperator  Operator===  OutDataTypeStr=boolean  RndMeth=Simplest  InputSameDT=off
  For Iterator : ForIterator  IterationLimit=Len  IndexMode=Zero-based
  Selector : Selector  IndexMode=Zero-based  InputPortWidth=Len  IndexOptions=Index vector (port)  Indices=[1 3]  OutputSizes=1
  Switch : Switch  Criteria=u2 ~= 0  SaturateOnIntegerOverflow=off  InputSameDT=off
  wires:
  Assignment/1 -> Data Store Write/1
  For Iterator/1 -> Selector/2, Assignment/3, Equal/1
  index/1 -> Equal/2
  Data Store Read1/1 -> Assignment/1, Selector/1
  Constant/1 -> Switch/1
  Equal/1 -> Switch/2
  Selector/1 -> Switch/3
  Switch/1 -> Assignment/2

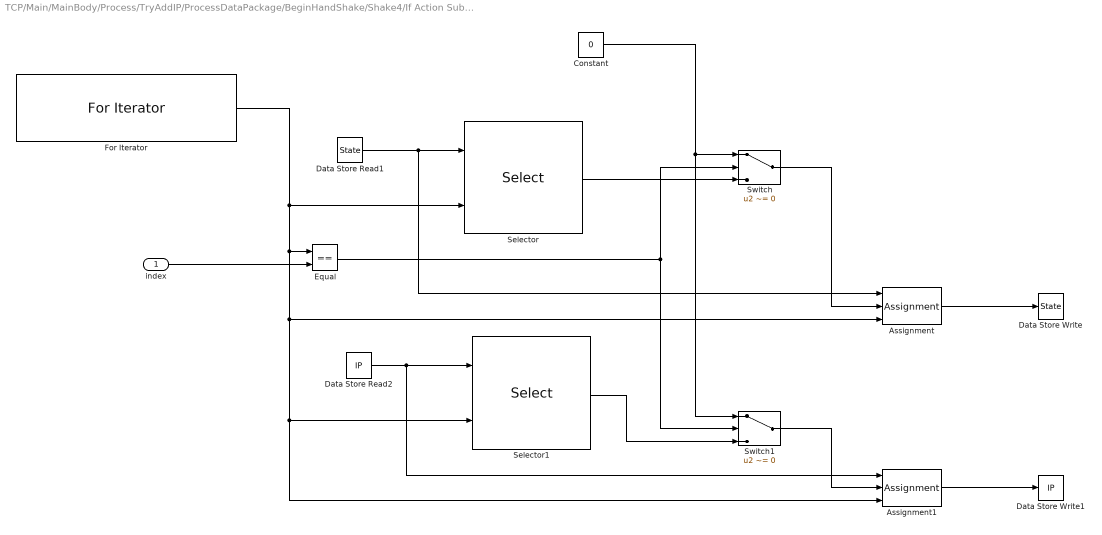
== system TCP/Main/MainBody/Process/TryAddIP/ProcessDataPackage/BeginHandShake/Shake4/If Action Subsystem/For Iterator Subsystem ==
  index : Inport
  Assignment : Assignment  IndexMode=Zero-based  DiagnosticForDimensions=Warning  IndexOptions=Index vector (port)  Indices=1  OutputSizes=1
  Assignment1 : Assignment  IndexMode=Zero-based  DiagnosticForDimensions=Warning  IndexOptions=Index vector (port)  Indices=1  OutputSizes=1
  Constant : Constant  Value=0  OutDataTypeStr=int32
  Data Store Read1 : DataStoreRead  DataStoreName=State  IndexOptions=Index vector (dialog)  Indices=1  OutputSizes=1
  Data Store Read2 : DataStoreRead  DataStoreName=IP  IndexOptions=Index vector (dialog)  Indices=1  OutputSizes=1
  Data Store Write : DataStoreWrite  DataStoreName=State  IndexOptions=Index vector (dialog)  Indices=1  OutputSizes=1
  Data Store Write1 : DataStoreWrite  DataStoreName=IP  IndexOptions=Index vector (dialog)  Indices=1  OutputSizes=1
  Equal : RelationalOperator  Operator===  OutDataTypeStr=boolean  RndMeth=Simplest  InputSameDT=off
  For Iterator : ForIterator  IterationLimit=Len  IndexMode=Zero-based
  Selector : Selector  IndexMode=Zero-based  InputPortWidth=Len  IndexOptions=Index vector (port)  Indices=[1 3]  OutputSizes=1
  Selector1 : Selector  IndexMode=Zero-based  InputPortWidth=Len  IndexOptions=Index vector (port)  Indices=[1 3]  OutputSizes=1
  Switch : Switch  Criteria=u2 ~= 0  SaturateOnIntegerOverflow=off  InputSameDT=off
  Switch1 : Switch  Criteria=u2 ~= 0  SaturateOnIntegerOverflow=off  InputSameDT=off
  wires:
  Assignment/1 -> Data Store Write/1
  For Iterator/1 -> Selector/2, Selector1/2, Assignment1/3, Assignment/3, Equal/1
  index/1 -> Equal/2
  Data Store Read1/1 -> Assignment/1, Selector/1
  Constant/1 -> Switch1/1, Switch/1
  Equal/1 -> Switch1/2, Switch/2
  Selector/1 -> Switch/3
  Switch/1 -> Assignment/2
  Data Store Read2/1 -> Assignment1/1, Selector1/1
  Assignment1/1 -> Data Store Write1/1
  Switch1/1 -> Assignment1/2
  Selector1/1 -> Switch1/3
